simulink model "controllore_simulink"  (Simulink 8.3)
settings: Solver=ode45  StartTime=0.0  StopTime=30  RelTol=1e-3
values from neighbouring files (symbols this model uses):
  A = 9    [controllore.m]
  Dp = 10^-3    (= 0.001)    [controllore.m]
  Tp = 1    [controllore.m]
  wp = 30    [controllore.m]
libraries: cstblocks x2
settings Model: Creator=matdo  LastModifiedBy=matdo
settings DataIOCC: SignalLoggingSaveFormat=Dataset
settings DebuggingCC: UnderspecifiedInitializationDetection=Simplified  StateNameClashWarn=none
settings GRTTargetCC: CombineOutputUpdateFcns=on  GRTInterface=off

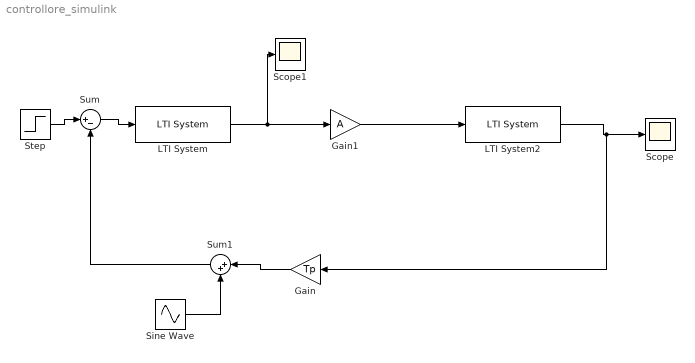
== system controllore_simulink ==
  Gain : Gain  Gain=Tp
  Gain1 : Gain  Gain=A
  LTI System : cstblocks/LTI System  sys=Ci  IC=[]
  LTI System2 : cstblocks/LTI System  sys=Gp  IC=[]
  Scope : Scope
  Scope1 : Scope
  Sine Wave : Sin  Amplitude=Dp  Frequency=wp  SampleTime=0
  Step : Step  Time=0  SampleTime=0
  Sum : Sum  Inputs=|+-
  Sum1 : Sum  Inputs=|++
  wires:
  LTI System/1 -> Scope1/1, Gain1/1
  Gain1/1 -> LTI System2/1
  Step/1 -> Sum/1
  Sum/1 -> LTI System/1
  LTI System2/1 -> Gain/1, Scope/1
  Gain/1 -> Sum1/1
  Sum1/1 -> Sum/2
  Sine Wave/1 -> Sum1/2
